simulink model "FnctnArch"  (R2023b)
settings: Solver=VariableStepAuto  StartTime=0.0  StopTime=10.0  RelTol=1e-3
settings Model: Creator=monis  LastModifiedBy=monis

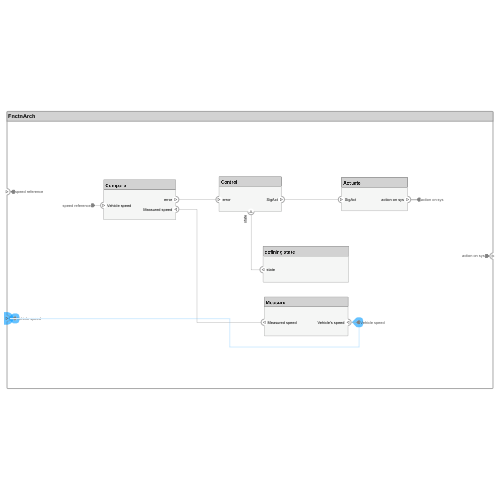
[thumbnail: Simulink's stored preview of the top-level diagram]
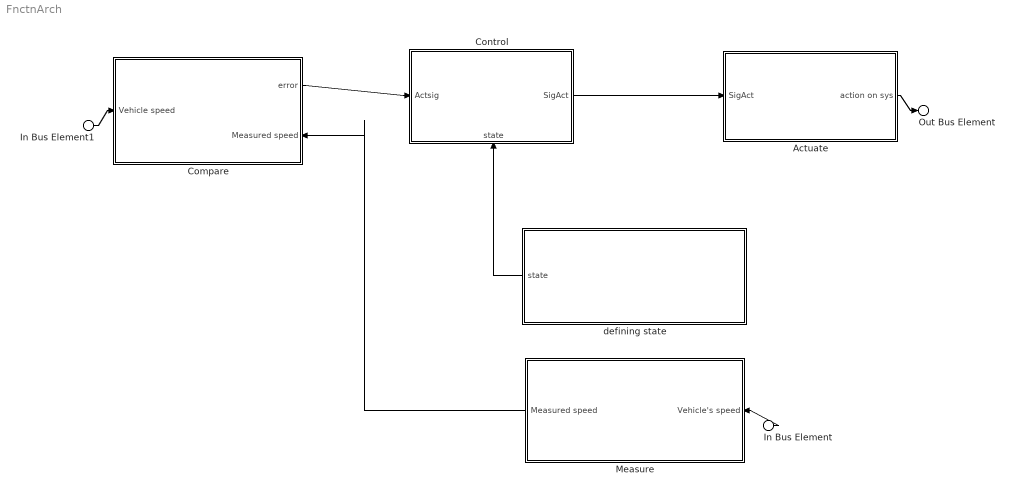
== system FnctnArch ==
  In Bus Element1 : Inport  PortName=speed reference
  In Bus Element : Inport  Port=2  PortName=Vehicle speed
  Actuate : Subsystem
      settings: PortSchema="{\"entries\":[{\"content\":{\"headerSize\":26,\"margin\":15,\"minimumSpacing\":25,\"sides\":[{\"content\":{\"connectorIds\":[\"In1\"]},\"type\":\"ConnectorPlacement.EquallySpacedRectSide\",\"uuid\":\"ada155ff-093c-4f64-a32a-d686ea6498a4\"},{\"content\":{\"connectorIds\":[\"Out1\"],\"side\":\"RIGHT\"},\"type\":\"ConnectorPlacement.EquallySpacedRectSide\",\"uuid\":\"9cdc1e9b-432d-4008-995c-5248d03da22f\"},{\"content\":{\"side\":\"TOP\"},\"type\":\"ConnectorPlacement.EquallySpacedRectSide\",\"uuid\":\"4d6e4fd0-71df-4c7a-8e23-78cd31fae1cd\"}]},\"type\":\"ConnectorPlacement.EquallySpacedConnector\",\"uuid\":\"e0804e1f-5645-4c9c-a0b7-54b4ff28d8a8\"}],\"packageUris\":[\"http://schema.mathworks.com/mf0/Connector/R2020b\"],\"version\":\"1.0\"}"
  Compare : Subsystem
      settings: PortSchema="{\"entries\":[{\"content\":{\"headerSize\":26,\"margin\":15,\"minimumSpacing\":25,\"sides\":[{\"content\":{\"connectorIds\":[\"In2\"]},\"type\":\"ConnectorPlacement.EquallySpacedRectSide\",\"uuid\":\"ada155ff-093c-4f64-a32a-d686ea6498a4\"},{\"content\":{\"connectorIds\":[\"Out1\",\"In1\"],\"side\":\"RIGHT\"},\"type\":\"ConnectorPlacement.EquallySpacedRectSide\",\"uuid\":\"9cdc1e9b-432d-4008-995c-5248d03da22f\"},{\"content\":{\"side\":\"TOP\"},\"type\":\"ConnectorPlacement.EquallySpacedRectSide\",\"uuid\":\"4d6e4fd0-71df-4c7a-8e23-78cd31fae1cd\"}]},\"type\":\"ConnectorPlacement.EquallySpacedConnector\",\"uuid\":\"e0804e1f-5645-4c9c-a0b7-54b4ff28d8a8\"}],\"packageUris\":[\"http://schema.mathworks.com/mf0/Connector/R2020b\"],\"version\":\"1.0\"}"
  Control : Subsystem
      settings: PortSchema="{\"entries\":[{\"content\":{\"headerSize\":26,\"margin\":15,\"minimumSpacing\":25,\"sides\":[{\"content\":{\"connectorIds\":[\"In2\"]},\"type\":\"ConnectorPlacement.EquallySpacedRectSide\",\"uuid\":\"ada155ff-093c-4f64-a32a-d686ea6498a4\"},{\"content\":{\"connectorIds\":[\"Out1\"],\"side\":\"RIGHT\"},\"type\":\"ConnectorPlacement.EquallySpacedRectSide\",\"uuid\":\"9cdc1e9b-432d-4008-995c-5248d03da22f\"},{\"content\":{\"side\":\"TOP\"},\"type\":\"ConnectorPlacement.EquallySpacedRectSide\",\"uuid\":\"4d6e4fd0-71df-4c7a-8e23-78cd31fae1cd\"},{\"content\":{\"connectorIds\":[\"In1\"],\"side\":\"BOTTOM\"},\"type\":\"ConnectorPlacement.EquallySpacedRectSide\",\"uuid\":\"f7133d39-cee6-4f54-9a48-2dff71677d6d\"}]},\"type\":\"ConnectorPlacement.EquallySpacedConnector\",\"uuid\":\"e0804e1f-5645-4c9c-a0b7-54b4ff28d8a8\"}],\"packageUris\":[\"http://schema.mathworks.com/mf0/Connector/R2020b\"],\"version\":\"1.0\"}"
  Measure : Subsystem
      settings: PortSchema="{\"entries\":[{\"content\":{\"headerSize\":26,\"margin\":15,\"minimumSpacing\":25,\"sides\":[{\"content\":{\"connectorIds\":[\"Out1\"]},\"type\":\"ConnectorPlacement.EquallySpacedRectSide\",\"uuid\":\"ada155ff-093c-4f64-a32a-d686ea6498a4\"},{\"content\":{\"connectorIds\":[\"In1\"],\"side\":\"RIGHT\"},\"type\":\"ConnectorPlacement.EquallySpacedRectSide\",\"uuid\":\"9cdc1e9b-432d-4008-995c-5248d03da22f\"},{\"content\":{\"side\":\"TOP\"},\"type\":\"ConnectorPlacement.EquallySpacedRectSide\",\"uuid\":\"4d6e4fd0-71df-4c7a-8e23-78cd31fae1cd\"}]},\"type\":\"ConnectorPlacement.EquallySpacedConnector\",\"uuid\":\"e0804e1f-5645-4c9c-a0b7-54b4ff28d8a8\"}],\"packageUris\":[\"http://schema.mathworks.com/mf0/Connector/R2020b\"],\"version\":\"1.0\"}"
  defining state : Subsystem
      settings: PortSchema="{\"entries\":[{\"content\":{\"headerSize\":26,\"margin\":15,\"minimumSpacing\":25,\"sides\":[{\"content\":{\"connectorIds\":[\"Out1\"]},\"type\":\"ConnectorPlacement.EquallySpacedRectSide\",\"uuid\":\"ada155ff-093c-4f64-a32a-d686ea6498a4\"},{\"content\":{\"side\":\"RIGHT\"},\"type\":\"ConnectorPlacement.EquallySpacedRectSide\",\"uuid\":\"9cdc1e9b-432d-4008-995c-5248d03da22f\"},{\"content\":{\"side\":\"TOP\"},\"type\":\"ConnectorPlacement.EquallySpacedRectSide\",\"uuid\":\"4d6e4fd0-71df-4c7a-8e23-78cd31fae1cd\"}]},\"type\":\"ConnectorPlacement.EquallySpacedConnector\",\"uuid\":\"e0804e1f-5645-4c9c-a0b7-54b4ff28d8a8\"}],\"packageUris\":[\"http://schema.mathworks.com/mf0/Connector/R2020b\"],\"version\":\"1.0\"}"
  Out Bus Element : Outport  PortName=action on sys
  wires:
  Measure/1(Measured speed) -> Compare/1(Measured speed)
  In Bus Element1/1 -> Compare/2(Vehicle speed)
  Actuate/1(action on sys) -> Out Bus Element/1
  Control/1(SigAct) -> Actuate/1(SigAct)
  Compare/1(error) -> Control/2(Actsig)
  defining state/1(state) -> Control/1(state)
  In Bus Element/1 -> Measure/1(Vehicle's speed)

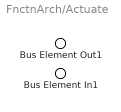
== system FnctnArch/Actuate ==
  Bus Element In1 : Inport  PortName=SigAct
  Bus Element Out1 : Outport  PortName=action on sys

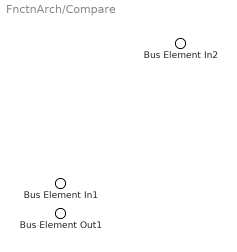
== system FnctnArch/Compare ==
  Bus Element In2 : Inport  PortName=Measured speed
  Bus Element In1 : Inport  Port=2  PortName=Vehicle speed
  Bus Element Out1 : Outport  PortName=error

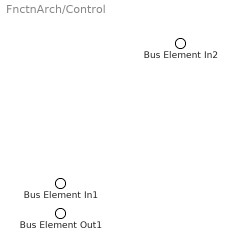
== system FnctnArch/Control ==
  Bus Element In2 : Inport  PortName=state
  Bus Element In1 : Inport  Port=2  PortName=Actsig
  Bus Element Out1 : Outport  PortName=SigAct

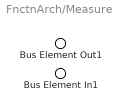
== system FnctnArch/Measure ==
  Bus Element In1 : Inport  PortName=Vehicle's speed
  Bus Element Out1 : Outport  PortName=Measured speed

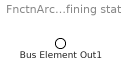
== system FnctnArch/defining state ==
  Bus Element Out1 : Outport  PortName=state
